simulink model "Adaptive_CT_ur10v"  (R2021b)
(part 18 of 20)

et24 = qd5.*(t1268.*-2.0-t1270.*2.0-t1739-t1742-t1788+t1823.*2.0+t1850-t1857-t1892+t2037+t2044+t2172+t2187+t2198+t2203+t8.*(t599+t612-t986-t1082-t1084+t449.*(t60-t190).*8.084033333333334e-4)+t2.*(t600+t610-t997-t1068-t1069+t451.*(t61-t239).*8.084033333333334e-4))-qd2.*(t2193+t2199+t1495.*t1680+t15.*t942.*t953+t17.*t942.*t953);
et25 = t1397-t1784-t1812+t1862+t1876-t1911-t1947-t2042-t2101+t2109+t2117+t2134+t2135-t2178+t2293+t2311+(t1321.*(t261+t455-t955-t1023))./2.0+t132.*(t600+t610-t997-t1068-t1069+t451.*(t61-t239).*8.084033333333334e-4)+t171.*(t599+t612-t986-t1082-t1084+t449.*(t60-t190).*8.084033333333334e-4);
et26 = t2.*t942.*(t441-t442-t647+t1012)+(t8.*t25.*(-t681+t1059.*(t61-t239).*8.084033333333334e-4+t341.*(t289-t476+t171.*(t60-t190)).*8.084033333333334e-4))./2.0;
et27 = (t8.*t29.*(t633-t852+t1418+t1752+t1545.*(t61-t239).*8.084033333333334e-4+t252.*(t289-t476+t171.*(t60-t190)).*8.084033333333334e-4))./2.0+t2.*t491.*(t426-t1001)+t8.*t491.*(t443-t1013);
et28 = t1546+t1549-t1588-t1988+t2063+t2072-t2139-t2141-t2176+t2225+t2283+t2286-t789.*t1680+(t25.*(t703+t979-t1289-t1291+t192.*(-t268-t292+t331+t334+t393+t2.*t25.*(t60-t190)).*8.084033333333334e-4+t236.*(-t267-t293+t348+t352+t382+t8.*t25.*(t61-t239)).*8.084033333333334e-4))./2.0;
et29 = t2.*t29.*(t599+t612-t986-t1082-t1084+t449.*(t60-t190).*8.084033333333334e-4)-t8.*t902.*t942-t2.*t914.*t942+(t8.*t25.*(t791+t1331+t935.*(t61-t239).*8.084033333333334e-4))./2.0;
et30 = t2331+qd4.*(t1643+t1644+t1732+t1782+t1841+t1843+t1991+t2001-t2008+t2035+t2041+t2171+t2183+t2196+t2202-t2223+t2275+t2279)+qd3.*(t1712+t1715+t1782+t1841+t1843+t1844+t2020+t2026+t2035+t2041-t2166+t2171+t2183+t2196+t2202+t2275+t2279);
et31 = -qd1.*(t713+t983-t1288-t1290-t1709+t1717-t2087-t2093+t192.*(-t268-t292+t331+t334+t393+t2.*t25.*(t60-t190)).*4.042016666666667e-4+t236.*(-t267-t293+t348+t352+t382+t8.*t25.*(t61-t239)).*4.042016666666667e-4)+qd2.*(t1739+t1742+t1782+t1841+t1843+t1892+t2040+t2046+t2171+t2185+t2196+t2202+t2275+t2279)+qd5.*(et28+et29);
et32 = t127+t220+t228+t255+t264-qd2.*(et23+et24)+qd3.*(-t2324+qd5.*(t1212+t1213+t1268+t1270+t1712+t1715+t1788+t1799+t1831+t1844+t1853+t1857+t2023+t2028+t2166+t2173+t2201+t2204+t2217+t2218)+qd4.*(t1428+t1430+t1434+t1436+t1454+t1458+t1884+t1923+t2151+t2152+t2193+t2199)+qd1.*(t540+t977+t1007+t1086+t1095-t1487+t1489+t1586+t1587)+qd2.*(t1507+t1513+t1514+t1515+t2080+t2083+t2193+t2199)+qd3.*(t2193+t2199+t1395.*t1680+t15.*t904.*t942+t17.*t904.*t942))+qdd3.*t2319+qdd4.*t2321;
et33 = qd6.*(t2328+qd2.*(t1710+t1719+t1783+t1789+t1840+t1859+t1969+t1975+t2030+t2170+t2205+t2210+t2306+t2310)+qd4.*(t1570+t1617+t1625+t1783+t1840+t1859-t1894+t1914+t1922+t1956+t1965+t2029+t2125+t2170+t2205+t2210+t2306+t2310)+qd1.*(t623+t778+t1383+t1390+t1670+t1721+t1735+t2021+t2025+(t915.*(t443-t1013))./2.0)-qd5.*(et25+et26+et27)+qd3.*(t1662+t1676+t1770+t1783+t1840+t1859+t1934+t1941+t1956+t1965+t1987+t2029+t2170+t2205+t2210+t2306+t2310))+qdd1.*(t542+t1077+t1105+t1591+t1592)+qdd2.*(t1821+t1822+t15.*t956+t17.*t956+t1680.^2);
et34 = -qd1.*(qd4.*(-t1304+t1306+t1424-t1427+t1537+t1540+t1955+t1959+t2165)+qd3.*(-t1465+t1468+t1487-t1489+t1586+t1587+t1955+t1959+t2165)-qd1.*(t243+t755+t757-t915.*t1099+t917.*t1101)+qd2.*(t1506+t1517+t1608+t1609+t1955+t1959+t2165)-qd6.*(t1218-t1433+t1554+t1670+t2000-t2002+t2021+t2025+(t915.*(t443-t1013))./2.0+(t29.*t30.*(t329+t834+t236.*(t61-t239).*8.084033333333334e-4))./2.0)+qd5.*(t1168+t1170+t1206+t1380+t1385+t1419+t1548+t1556+t1709+t1718+t1974+t1983+t2087+t2093+t2174));
et35 = qd4.*(qd3.*(t1426+t1429+t1435+t1437+t1454+t1458+t2126+t2149+t2151+t2193+t2199)+qd4.*(t1454+t1458+t1923+t2049+t2193+t2199-t1648.*t1792)+qd5.*(t1139+t1140+t1268+t1270+t1643+t1644+t1788+t1831+t1853+t1857+t1942+t1996+t2004+t2008+t2173+t2201+t2204+t2217+t2218+t2223)-qd6.*(t1617+t1625+t1790+t1856+t1861+t1894+t1913+t1921+t2124+t2175+t2209+t2212)+qd1.*(t540+t977+t1007+t1086+t1095-t1424+t1427+t1537+t1540)+qd2.*(t1463+t1467+t1469+t1470+t2155+t2157+t2193+t2199))+qdd6.*(t1683+t1700+t1785+t1869+t1871+t1900)-qdd5.*(t1726+t1728+t1786+t1842+t1846+t2018)-qd5.*(et30+et31);
et36 = t220-qdd1.*t981+qdd2.*t1802+qd2.*(t999+qd3.*(t452+t459-t1090-t1216+t15.*t20.*t22.*1.63763645e-1+t17.*t20.*t22.*1.63763645e-1)+qd2.*(t1066-t812.*(t2.*(t296-t2.*t9.*(1.53e+2./2.5e+2))+t8.*(t299-t8.*t9.*(1.53e+2./2.5e+2)))+t178.*t274+t179.*t274-t568.*t980))+qdd3.*(t211+t212+t15.*t31.*3.2752729e-1+t17.*t31.*3.2752729e-1+t980.^2);
et37 = qd3.*(t999+qd2.*(-t452-t459+t1090+t1216-t980.*(t2.*(t296-t2.*t9.*(1.53e+2./2.5e+2))+t8.*(t299-t8.*t9.*(1.53e+2./2.5e+2))).*2.0+t15.*t20.*t22.*4.91290935e-1+t17.*t20.*t22.*4.91290935e-1)+qd3.*(-t1193+t15.*t20.*t22.*3.2752729e-1+t17.*t20.*t22.*3.2752729e-1))-qd1.*(t1000+qd2.*t988-qd1.*(t151.*t400+t177.*t406));
et38 = t220+t229+qdd1.*t1532+qdd2.*t2177+qdd4.*t2179+qd2.*(-qd3.*(t752+t754+t1704-(t948.*t1138)./2.0+(t15.*t342.*t351)./2.0+(t17.*t342.*t351)./2.0)+qd1.*(t883-t889+t989+t990)+qd4.*(t506+t508+t596+t597+t1346+t1480-t1779+t1803+t15.*t144.*t342+t17.*t144.*t342)+qd2.*(t1108.*t1138+t15.*t342.*t420+t17.*t342.*t420))+qdd3.*(t519+t521+t15.*t356+t17.*t356+t1138.^2);
et39 = -qd3.*(qd4.*(-t506-t508-t1346.*2.0+t1737+t1808+t15.*t29.*t342.*1.22925e-1+t17.*t29.*t342.*1.22925e-1)-qd1.*t1945-qd2.*(t752+t754+t1704+t948.*t1138.*(3.0./2.0)-t15.*t342.*t351.*(3.0./2.0)-t17.*t342.*t351.*(3.0./2.0))+qd3.*(-t948.*t1138+t15.*t342.*t351+t17.*t342.*t351))-qd4.*(qd2.*(t495+t498+t506+t508+t596+t597+t1779+t1798+t1803)+qd4.*(t495+t498+t1352+t1627+t1165.*(t936-t937))+qd3.*(t496+t499+t506+t508+t1738+t1803)-qd1.*(-t661+t664+t1411))-qd1.*(qd1.*(t487+t502.*t708-t513.*t702)+qd3.*t1945+qd2.*(t882-t883+t889+t897+t989+t990)+qd4.*(t661-t664+t1411));
et40 = qd3.*(t1179+t1300-t1301-t1332+t1729+t1734-t1845+t2168-t2242+t2243+t25.*(t527+t813)+t2.*t29.*(t551-t821)+t8.*t29.*(t552-t822)+(t8.*t481.*(t423-t716))./2.0)-qd1.*(t710+t729-t830-t969+t991-t1173+t1508+t1874+(t836.*(t423-t716))./2.0+(t1100.*(t421-t432-t619+t718))./2.0)+qd4.*(t1179+t1261+t1267+t1300-t1301+t1673+t1674+t1720-t1733+t1916-t2162+t2224-t2242+t2243+t25.*(t527+t813)+t8.*t479.*(t421-t432-t619+t718)+t2.*t29.*(t551-t821)+t8.*t29.*(t552-t822));
et41 = qd2.*(t1179+t1300-t1301-t1332+t1720+t1756+t1759-t1845-t2162+t2186-t2242+t2243+t25.*(t527+t813)+t8.*t479.*(t421-t432-t619+t718)+t2.*t29.*(t551-t821)+t8.*t29.*(t552-t822)+(t8.*t481.*(t423-t716))./2.0)-qd5.*(t1147+t1153+t1361+t1479+t1484+t1593+t1707+t1771+t1773+t1837+t1839+t2073+t2231+t2247+t2248-t790.*t1603-t8.*t479.*t602+t2.*t479.*(t241-t419));
et42 = t220+t228+t256+t265-qd1.*(qd4.*(t527+t813+t952+t966+t1091-t1093+t1316+t1318+t1706+t1708)+qd1.*(t235+t525+t549-t829.*t1102+t836.*t1100)-qd3.*(t1159+t1166+t1169+t1384+t1386+t1705+t1711)-qd2.*(t1159+t1208+t1215-t1220+t1225+t1384+t1386+t1705+t1711)+qd5.*(t776+t787-t802+t806+t1070-t1131-t1187-t1189-t1251-t1252+t1508-t1724-t1725+t1874+(t836.*(t423-t716))./2.0+(t1100.*(t421-t432-t619+t718))./2.0))+qd5.*(et40+et41);
et43 = -qd3.*(qd2.*(t993+t995+t1202+t1211+t2084-t1396.*t1603.*(3.0./2.0)-t15.*t479.*t481.*(3.0./2.0)-t17.*t479.*t481.*(3.0./2.0))+qd4.*(t794.*(3.0./2.0)+t796.*(3.0./2.0)+t824+t826+t1202+t1211-t1885.*2.0+t2103+t2150)-qd5.*(t1192+t1201+t1234+t1236+t1313+t1320+t1332+t1333+t1456+t1457+t1730+t1731-t1797.*2.0+t1845+t2167+t6.*t15.*t130.*t479+t6.*t17.*t130.*t479)-qd3.*(t1203+t1209+t1396.*t1603+t15.*t479.*t481+t17.*t479.*t481)+qd1.*(t553+t798+t1166+t1169+t1384+t1386))+qdd2.*t2264+qdd4.*t2269;
et44 = qd2.*(qd3.*(t993+t995+t1203+t1209+t2084+(t1396.*t1603)./2.0+(t15.*t479.*t481)./2.0+(t17.*t479.*t481)./2.0)+qd5.*(t669+t672+t723+t726+t1192+t1201+t1234+t1236+t1313+t1320+t1332+t1333+t1456+t1457+t1756+t1759+t1800+t1832+t1845+t2186)-qd1.*(t553+t798-t1215+t1220+t1384+t1386)-qd4.*(t794+t796+t824+t826+t907+t908+t1202+t1211+t1886+t1925+t2133+t2150)+qd2.*(t1203+t1209+t1496.*t1603+t15.*t479.*t581+t17.*t479.*t581))+qdd3.*(t1277+t1278+t15.*t497+t17.*t497+t1603.^2)+qdd5.*(t1302-t1303-t1319-t1961+t25.*(t530-t803)+t8.*t479.*(t423-t716))+qdd1.*(t1160+t1353+t1358);
et45 = qd4.*(-qd4.*(t794+t796+t1202+t1211+t1886+t2052+t1535.*t1793)+qd5.*(t558+t560+t669+t672+t1192+t1201+t1234+t1236+t1271+t1275+t1313+t1320+t1456+t1457+t1673+t1674+t1800+t1916+t1943+t2224)+qd1.*(t540+t814-t1091+t1093+t1316+t1318)+qd2.*(-t794-t796+t824+t826+t907+t908+t1203+t1209-t2133+t2144+t2150)+qd3.*(t824-t825+t826-t827+t1203+t1209+t2103+t2150));
et46 = t1397-t1784-t1812+t1862+t1876-t1896-t1947-t2042+t2085-t2101+t2109+t2134+t2135-t2178+t2293+t2311+(t1321.*(t261+t455-t955-t1023))./2.0+t132.*(t600+t610-t997-t1068-t1069+t451.*(t61-t239).*8.084033333333334e-4)+t171.*(t599+t612-t986-t1082-t1084+t449.*(t60-t190).*8.084033333333334e-4);
et47 = t2.*t890.*(t441-t442-t647+t1012)+(t8.*t25.*(-t681+t1059.*(t61-t239).*8.084033333333334e-4+t341.*(t289-t476+t171.*(t60-t190)).*8.084033333333334e-4))./2.0;
et48 = (t8.*t29.*(t633-t852+t1418+t1752+t1545.*(t61-t239).*8.084033333333334e-4+t252.*(t289-t476+t171.*(t60-t190)).*8.084033333333334e-4))./2.0+t2.*t491.*(t426-t1001)+t8.*t491.*(t443-t1013);
et49 = t2324+qd2.*(t1507+t1514+t2083+t2194+t2197-t1395.*t1602.*(3.0./2.0)-t15.*t890.*t904.*(3.0./2.0)-t17.*t890.*t904.*(3.0./2.0))-qd1.*(t540+t977+t1007+t1086+t1095+t1441+t1445+t1586+t1587)+qd4.*(t1407.*(-3.0./2.0)-t1409.*(3.0./2.0)+t1426+t1429-t1884.*2.0+t2102+t2149+t2194+t2197)-qd3.*(t2193+t2199+t1395.*t1602+t15.*t890.*t904+t17.*t890.*t904);
et50 = qd5.*(t1212.*-2.0-t1213.*2.0-t1712-t1715-t1788+t1796.*2.0-t1844+t1850-t1857+t2020+t2026-t2166+t2172+t2198+t2203+t8.*(t599+t612-t986-t1082-t1084+t449.*(t60-t190).*8.084033333333334e-4)+t2.*(t600+t610-t997-t1068-t1069+t451.*(t61-t239).*8.084033333333334e-4));
et51 = t1546+t1549-t1588-t1988+t2063+t2072-t2139-t2141-t2176+t2225+t2283+t2286-t789.*t1602+(t25.*(t703+t979-t1289-t1291+t192.*(-t268-t292+t331+t334+t393+t2.*t25.*(t60-t190)).*8.084033333333334e-4+t236.*(-t267-t293+t348+t352+t382+t8.*t25.*(t61-t239)).*8.084033333333334e-4))./2.0;
et52 = t2.*t29.*(t599+t612-t986-t1082-t1084+t449.*(t60-t190).*8.084033333333334e-4)-t8.*t890.*t902-t2.*t890.*t914+(t8.*t25.*(t791+t1331+t935.*(t61-t239).*8.084033333333334e-4))./2.0;
et53 = t2331+qd4.*(t1643+t1644+t1732+t1782+t1841+t1843-t1915+t1991+t2001+t2014+t2024+t2161+t2171+t2196+t2202-t2223+t2275+t2279)-qd1.*(t713+t983-t1288-t1290-t1652+t1661-t2087-t2093+t192.*(-t268-t292+t331+t334+t393+t2.*t25.*(t60-t190)).*4.042016666666667e-4+t236.*(-t267-t293+t348+t352+t382+t8.*t25.*(t61-t239)).*4.042016666666667e-4);
et54 = qd3.*(t1712+t1715+t1782+t1841+t1843+t1844+t2023+t2028+t2166+t2171+t2196+t2202+t2275+t2279)+qd2.*(t1712+t1715+t1782+t1841+t1843+t1844+t2014+t2024+t2037+t2044+t2161+t2171+t2187+t2196+t2202+t2275+t2279)+qd5.*(et51+et52);
et55 = t220+t228+t255+t264+qdd2.*t2319+qdd4.*t2320+qd6.*(t2328+qd3.*(t1662+t1676+t1770+t1783+t1840+t1859+t1933+t1936+t1985+t2170+t2205+t2210+t2306+t2310)+qd4.*(t1570+t1617+t1625+t1783-t1814+t1840+t1859+t1914+t1922+t1930+t1931+t1977+t2125+t2170+t2205+t2210+t2306+t2310)+qd1.*(t623+t778+t1383+t1390+t1628+t1721+t1735+t2021+t2025+(t835.*(t443-t1013))./2.0)-qd5.*(et46+et47+et48)+qd2.*(t1662+t1676+t1770+t1783+t1840+t1859+t1930+t1931+t1973+t1977+t1980+t2032+t2170+t2205+t2210+t2306+t2310))-qd3.*(et49+et50);
et56 = qd2.*(qd3.*(t1507+t1514+t2083+t2193+t2199+(t1395.*t1602)./2.0+(t15.*t890.*t904)./2.0+(t17.*t890.*t904)./2.0)+qd5.*(t1212+t1213+t1268+t1270+t1712+t1715+t1788+t1799+t1831+t1844+t1853+t1857+t2040+t2046+t2173+t2185+t2201+t2204+t2217+t2218)+qd4.*(t1407+t1409+t1434+t1436+t1463+t1470+t1884+t1923+t2136+t2152+t2193+t2199)-qd6.*(t1662+t1676+t1770+t1790+t1856+t1861+t1969+t1975+t2030+t2175+t2209+t2212)+qd1.*(t540+t977+t1007+t1086+t1095-t1482+t1483+t1586+t1587)+qd2.*(t2193+t2199+t1495.*t1602+t15.*t890.*t953+t17.*t890.*t953))+qdd1.*(t542+t1077+t1105+t1572+t1573)+qdd3.*(t1821+t1822+t15.*t909+t17.*t909+t1602.^2);
et57 = -qd1.*(qd4.*(-t1246+t1247+t1348-t1350+t1537+t1540+t1955+t1959+t2165)+qd2.*(-t1476+t1478+t1482-t1483+t1586+t1587+t1955+t1959+t2165)-qd1.*(t243+t755+t757+t828.*t1101-t835.*t1099)+qd3.*(t1441+t1445+t1586+t1587+t1955+t1959+t2165)-qd6.*(t1218-t1433+t1554+t1628+t2000-t2002+t2021+t2025+(t835.*(t443-t1013))./2.0+(t29.*t30.*(t329+t834+t236.*(t61-t239).*8.084033333333334e-4))./2.0)+qd5.*(t1125+t1132+t1206+t1380+t1385+t1419+t1548+t1556+t1652+t1669+t1974+t1983+t2087+t2093+t2174))-qd5.*(et53+et54);
et58 = qd4.*(qd2.*(t1407+t1409+t1426+t1429+t1472+t1474+t2136+t2143+t2149+t2193+t2199)+qd4.*(t1407+t1409+t1884+t2049+t2193+t2199-t1534.*t1792)+qd5.*(t1139+t1140+t1212+t1213+t1643+t1644+t1788+t1799+t1853+t1857+t1915+t1942+t1996+t2004+t2173+t2201+t2204+t2217+t2218+t2223)-qd6.*(t1617+t1625+t1790+t1814+t1856+t1861+t1913+t1921+t2124+t2175+t2209+t2212)+qd1.*(t540+t977+t1007+t1086+t1095-t1348+t1350+t1537+t1540)+qd3.*(t1426+t1428+t1429+t1430+t2102+t2149+t2193+t2199))+qdd6.*(t1642+t1653+t1785+t1852+t1869+t1871)-qdd5.*(t1685+t1688+t1786+t1842+t1846+t1960);
et59 = t229+qdd1.*t1415+qdd3.*t2179+qdd2.*t2213-qd4.*(t1439+qd2.*(t346+t355-t586-t589+t1491+t1638-t1375.*(t936-t937).*2.0)+qd4.*(t1627+t15.*t25.*t29.*6.7158025e-3+t17.*t25.*t29.*6.7158025e-3)+qd3.*(t346+t355+t509+t512+t1357+t1638-t1165.*(t936-t937).*2.0))+qd2.*(t1432-qd4.*(t345+t354+t586+t589-t1491+t1633)-qd3.*(t505+t507+t509+t512+t586+t589+t1357+t1491+t1778+t1795)+qd2.*(t1485+t213.*t420+t214.*t420+t1274.*t1375+t1108.*(t936-t937)));
et60 = -qd1.*(qd1.*(t487-t25.*t744.*8.195e-2+t163.*t708)+qd4.*t1411+qd3.*(t663+t668+t1411)+qd2.*(t742+t768+t1411))+qdd4.*(t519+t521+(t936-t937).^2+t15.*t35.*6.7158025e-3+t17.*t35.*6.7158025e-3)-qd3.*(t1439+qd4.*(t345+t354+t496+t499-t1357+t1633)+qd3.*(t505+t507+t1346+t1795-t1138.*t1165)+qd2.*(t496+t499+t505+t507+t596+t597+t1357+t1491+t1795+t1798));
et61 = qd4.*(t1179+t1261+t1267+t1300-t1301+t1672+t1743-t2224-t2242+t2243+t25.*(t527+t813)+(t8.*t361.*(t421-t432-t619+t718))./2.0+t2.*t29.*(t551-t821)+t8.*t29.*(t552-t822))-qd1.*(t710+t729-t830-t969+t991-t1173+t1359+t1874+(t575.*(t423-t716))./2.0+(t1100.*(t421-t432-t619+t718))./2.0)+qd3.*(t1179+t1261+t1267+t1300-t1301+t1656+t1730+t1731+t1741-t1907+t2167-t2220-t2242+t2243+t25.*(t527+t813)+t8.*t361.*(t421-t432-t619+t718)+t2.*t29.*(t551-t821)+t8.*t29.*(t552-t822));
et62 = qd2.*(t1179+t1261+t1267+t1300-t1301+t1656+t1741+t1756+t1759-t2006+t2186-t2220-t2242+t2243+t25.*(t527+t813)+t8.*t361.*(t421-t432-t619+t718)+t2.*t29.*(t551-t821)+t8.*t29.*(t552-t822))-qd5.*(t1147+t1153+t1361+t1479+t1484+t1593+t1707+t1771+t1773+t1837+t1839+t2073+t2231+t2247+t2248-t790.*t1793-t8.*t361.*t602+t2.*t361.*(t241-t419));
et63 = t228+t256+t265-qd1.*(qd3.*(t527+t813+t974-t975+t1072+t1081+t1316+t1318+t1706+t1708)+qd2.*(t527+t813-t1031+t1038+t1141+t1146+t1316+t1318+t1706+t1708)+qd1.*(t235+t525+t549+t575.*t1100-t577.*t1102)+qd5.*(t679+t685-t802+t806+t1070-t1131-t1187-t1189-t1251-t1252+t1359-t1724-t1725+t1874+(t575.*(t423-t716))./2.0+(t1100.*(t421-t432-t619+t718))./2.0)+qd4.*(t527+t813+t887+t895+t1316+t1318+t1706+t1708))+qdd3.*t2269+qdd2.*t2300;
et64 = qd3.*(qd3.*(t793+t795+t1203+t1209+t1886+t2146+t1535.*t1603)+qd5.*(t558+t560+t669+t672+t1192+t1201+t1234+t1236+t1271+t1275+t1313+t1320+t1456+t1457+t1730+t1731+t1741+t1800+t1943+t2167)+qd1.*(t540+t814-t974+t975+t1316+t1318)+qd2.*(t793+t795+t837+t838+t907+t908+t1203+t1209+t1890+t1929+t2144+t2146)-qd4.*(t696+t698+t825+t827+t1202+t1211+t1890+t2057))+qdd4.*(t1277+t1278+t15.*t377+t17.*t377+t1793.^2)-qd4.*(qd4.*(t1202+t1211+t2052+t15.*t361.*t368+t17.*t361.*t368)-qd5.*(t1192+t1201+t1234+t1236+t1271+t1275+t1313+t1320+t1456+t1457+t1673+t1674+t1741-t1939.*2.0+t2224+t6.*t15.*t130.*t361+t6.*t17.*t130.*t361)+qd3.*(t697+t699-t825-t827+t1202+t1211+t1888+t2055-t1535.*t1793.*2.0)+qd2.*(t697+t699-t907-t908+t1202+t1211+t1927+t2055-t1649.*t1793.*2.0)-qd1.*(t540+t814+t887+t895+t1316+t1318));
et65 = qdd1.*(t1160+t1298+t1299)+qd5.*(et61+et62)+qd2.*(qd5.*(t558+t560+t723+t726+t1192+t1201+t1234+t1236+t1271+t1275+t1313+t1320+t1456+t1457+t1741+t1756+t1759+t1832+t1943+t2186)+qd1.*(t540+t814+t1031-t1038+t1316+t1318)+qd2.*(t1203+t1209+t1925+t1496.*t1793+t1649.*t1681+t15.*t361.*t581+t17.*t361.*t581)+qd3.*(t793+t795+t825+t827+t911+t912+t1203+t1209+t1890+t1929+t2127+t2146)-qd4.*(t696+t698+t907+t908+t1202+t1211+t1929+t2057))-qdd5.*(t1178+t1239+t1244+t1303+t1309+t2119);
et66 = t1397-t1784-t1812+t1862-t1868+t1876-t1947-t2042-t2101+t2109+t2134+t2135+t2159-t2178+t2293+t2311+(t1321.*(t261+t455-t955-t1023))./2.0+t132.*(t600+t610-t997-t1068-t1069+t451.*(t61-t239).*8.084033333333334e-4)+t171.*(t599+t612-t986-t1082-t1084+t449.*(t60-t190).*8.084033333333334e-4);
et67 = t2.*t773.*(t441-t442-t647+t1012)+(t8.*t25.*(-t681+t1059.*(t61-t239).*8.084033333333334e-4+t341.*(t289-t476+t171.*(t60-t190)).*8.084033333333334e-4))./2.0;
et68 = (t8.*t29.*(t633-t852+t1418+t1752+t1545.*(t61-t239).*8.084033333333334e-4+t252.*(t289-t476+t171.*(t60-t190)).*8.084033333333334e-4))./2.0+t2.*t491.*(t426-t1001)+t8.*t491.*(t443-t1013);
et69 = t2327-qd4.*(t1576+t1617+t1625+t1783+t1840+t1859+t1913+t1921+t2124+t2170+t2205+t2210+t2306+t2310)+qd3.*(t1576-t1783-t1811-t1840+t1854-t1905+t1933+t1936+t1985-t2123-t2170-t2205+t2208+t2304+t2308+t8.*t773.*(t261+t455-t955-t1023)+(t2.*t785.*(t426-t1001))./2.0+(t8.*t785.*(t443-t1013))./2.0)+qd2.*(t1576-t1783-t1840+t1854-t1891-t1905+t1969+t1975+t2030-t2123-t2170-t2205+t2208+t2304+t2308+t8.*t773.*(t261+t455-t955-t1023)+(t2.*t785.*(t426-t1001))./2.0+(t8.*t785.*(t443-t1013))./2.0)-qd1.*(t623+t778+t1383+t1390+t1538+t1721+t1735+t2021+t2025+(t574.*(t443-t1013))./2.0);
et70 = qd5.*(et66+et67+et68);
et71 = t1546+t1549-t1588-t1988+t2063+t2072-t2139-t2141-t2176+t2225+t2283+t2286-t789.*t1792+(t25.*(t703+t979-t1289-t1291+t192.*(-t268-t292+t331+t334+t393+t2.*t25.*(t60-t190)).*8.084033333333334e-4+t236.*(-t267-t293+t348+t352+t382+t8.*t25.*(t61-t239)).*8.084033333333334e-4))./2.0;
et72 = t2.*t29.*(t599+t612-t986-t1082-t1084+t449.*(t60-t190).*8.084033333333334e-4)-t8.*t773.*t902-t2.*t773.*t914+(t8.*t25.*(t791+t1331+t935.*(t61-t239).*8.084033333333334e-4))./2.0;
et73 = t2331+qd3.*(t1643+t1644-t1740+t1782+t1841+t1843+t1906+t1989+t1999+t2020+t2026-t2166+t2171+t2196+t2202+t2219+t2275+t2279)-qd1.*(t713+t983-t1288-t1290-t1574+t1580-t2087-t2093+t192.*(-t268-t292+t331+t334+t393+t2.*t25.*(t60-t190)).*4.042016666666667e-4+t236.*(-t267-t293+t348+t352+t382+t8.*t25.*(t61-t239)).*4.042016666666667e-4);
et74 = qd4.*(t1643+t1644+t1740+t1782+t1841+t1843+t1996+t2004+t2171+t2196+t2202+t2223+t2275+t2279)+qd2.*(t1643+t1644-t1740+t1782+t1841+t1843+t1989+t1999+t2005+t2037+t2044+t2171+t2187+t2196+t2202+t2219+t2275+t2279)+qd5.*(et71+et72);
et75 = -qd4.*(t2049+t2193+t2199+t15.*t773.*t785+t17.*t773.*t785)+qd3.*(t1343+t1344+t1428+t1430+t1887+t2054+t2194+t2197-t1534.*t1792.*2.0)+qd2.*(t1343+t1344+t1463+t1470+t1926+t2054+t2194+t2197-t1648.*t1792.*2.0);
et76 = qd5.*(t1139.*-2.0-t1140.*2.0+t1646+t1650-t1740-t1788+t1850-t1857+t1938.*2.0+t1991+t2001+t2172+t2198+t2203-t2223+t8.*(t599+t612-t986-t1082-t1084+t449.*(t60-t190).*8.084033333333334e-4)+t2.*(t600+t610-t997-t1068-t1069+t451.*(t61-t239).*8.084033333333334e-4))-qd1.*(t540+t977+t1007+t1086+t1095+t1176+t1181+t1537+t1540);
et77 = qd6.*(t1576+t1617+t1625+t1790+t1856+t1861+t1913+t1921+t2124+t2175+t2209+t2212);
et78 = t228+t255+t264-qd6.*(et69+et70)+qd2.*(qd5.*(t1139+t1140+t1268+t1270+t1643+t1644+t1740+t1788+t1831+t1853+t1857+t1942+t2040+t2046+t2173+t2185+t2201+t2204+t2217+t2218)+qd3.*(t1405+t1408+t1435+t1437+t1463+t1470+t1889+t1928+t2126+t2145+t2193+t2199)-qd6.*(t1576+t1617+t1625+t1790+t1856+t1861+t1969+t1975+t2030+t2175+t2209+t2212)+qd1.*(t540+t977+t1007+t1086+t1095-t1315+t1317+t1537+t1540)+qd4.*(t1339+t1341+t1463+t1470+t1926+t2054+t2193+t2199)+qd2.*(-t1923+t2193+t2199+t1495.*t1792+t1648.*t1680+t15.*t773.*t953+t17.*t773.*t953))+qdd2.*t2321+qdd3.*t2320-qd5.*(et73+et74)+qdd1.*(t542+t1077+t1105+t1522+t1523)+qdd4.*(t1821+t1822+t15.*t777+t17.*t777+t1792.^2);
et79 = -qd1.*(qd3.*(t1262-t1265-t1337+t1338+t1537+t1540+t1955+t1959+t2165)+qd2.*(t1315-t1317-t1402+t1406+t1537+t1540+t1955+t1959+t2165)-qd1.*(t243+t755+t757-t574.*t1099+t576.*t1101)+qd4.*(t1176+t1181+t1537+t1540+t1955+t1959+t2165)-qd6.*(t1218-t1433+t1538+t1554+t2000-t2002+t2021+t2025+(t574.*(t443-t1013))./2.0+(t29.*t30.*(t329+t834+t236.*(t61-t239).*8.084033333333334e-4))./2.0)+qd5.*(t1039+t1049+t1206+t1380+t1385+t1419+t1548+t1556+t1574+t1582+t1974+t1983+t2087+t2093+t2174))-qd4.*(et75+et76+et77);
et80 = qd3.*(qd5.*(t1139+t1140+t1212+t1213+t1643+t1644+t1740+t1788+t1799+t1853+t1857+t1942+t2023+t2028+t2166+t2173+t2201+t2204+t2217+t2218)+qd3.*(t1405+t1408-t1884+t2145+t2193+t2199+t1534.*t1602)+qd2.*(t1405+t1408+t1428+t1430+t1472+t1474+t1889+t1928+t2143+t2145+t2193+t2199)-qd6.*(t1576+t1617+t1625+t1790+t1856+t1861+t1933+t1936+t1985+t2175+t2209+t2212)+qd1.*(t540+t977+t1007+t1086+t1095-t1262+t1265+t1537+t1540)+qd4.*(t1339+t1341+t1428+t1430+t1887+t2054+t2193+t2199))+qdd6.*(t1610+t1616+t1785+t1869+t1871+t2013)-qdd5.*(t1631+t1634+t1786+t1842+t1846+t2118);
et81 = qd4.*(-t919+t1148+t1154+t1599+t1613+t1615+t1692+t1766+t1767+t1838+t1849-t1979+t2075+t2227+t2245+t2246+(t2.*t361.*(t241-t419))./2.0)+qd3.*(-t1003+t1148+t1154+t1599+t1613+t1615+t1692+t1766+t1767-t1817+t1838+t1849+t2075+t2227+t2245+t2246+(t2.*t479.*(t241-t419))./2.0)+qd2.*(-t1065+t1148+t1154+t1599+t1613+t1615+t1692+t1766+t1767+t1838+t1849-t1865+t2075+t2227+t2245+t2246+(t2.*t580.*(t241-t419))./2.0);
et82 = -qd1.*(t1256+t1259+t1452+t1461+t6.*t29.*t624.*5.077704166666666e-4+t12.*t29.*t622.*5.077704166666666e-4)+qd5.*(t25.*(t972+t973).*(-1.0./2.0)-t790.*t1264+t1036.*(t241-t419)+t602.*(t423-t716)+(t8.*t29.*t1597)./2.0+(t2.*t29.*(t1026-t1043))./2.0);
et83 = qd1.*(t12.*t68.*1.015540833333333e-3+t371.*t1100+t380.*t1102)+qd5.*(t972+t973+t1256+t1259+t1452+t1461-t12.*t25.*t68.*1.015540833333333e-3+(t2.*t29.*t1097)./2.0+(t8.*t29.*(t614-t638))./2.0)+qd4.*(t693+t695+t711+t712-t831-t970+t982+t1129+t1130-t1174+t1196+t1198+t1349+t1863+t575.*(t423-t716)+t1100.*(t421-t432-t619+t718))-qd3.*(-t809-t818+t1133+t1134+t1188+t1190+t1502+t1505+t1866+t1872+t2216);
et84 = -qd2.*(-t891-t898+t1133+t1134+t1188+t1190+t1551+t1553+t1866+t1872+t2216);
et85 = -qd4.*(qd4.*(t558+t560+t1255+t1260+t1464+t1466+t1659+t1668+t1733+t1943+t2220+t2240+t2241)-qd5.*(t919+t924+t1157+t1161+t1379+t1490+t1492+t1595+t1611+t1612+t1979)+qd3.*(t559+t561+t670+t673+t1255+t1260+t1464+t1466+t1659+t1668+t1810+t1907+t1954+t2220+t2240+t2241)+qd2.*(t559+t561+t724+t727+t1255+t1260+t1464+t1466+t1659+t1668+t1848+t1954+t2006+t2220+t2240+t2241)-qd1.*(t693+t695+t805+t815+t1196+t1198))-qd3.*(qd3.*(t669+t672+t1323+t1325+t1464+t1466+t1723+t1727+t1800+t1826+t2162+t2240+t2241)-qd5.*(t1003+t1015+t1157+t1161+t1379+t1490+t1492+t1595+t1611+t1612+t1817)+qd4.*(t559+t561+t670+t673+t1255+t1260+t1464+t1466+t1723+t1727+t1733+t1810+t1954+t2162+t2240+t2241)+qd2.*(t670+t673+t724+t727+t1323+t1325+t1464+t1466+t1723+t1727+t1810+t1826+t1848+t2162+t2240+t2241)-qd1.*(t805+t809+t815+t818+t1196+t1198))-t6.*t29.*5.675085e-1;
et86 = -qdd3.*(t1319+t1322+t1748+t1757+t1961)-qdd4.*(t1239+t1244+t1748+t1757+t2119)-qdd2.*(t1356+t1360+t1748+t1757+t2019)-qdd1.*(t1620+t1623+t1658)+qdd5.*((t423-t716).^2+t25.*t1658+t1036.^2+t1264.^2+t2.*t29.*t1744+t8.*t29.*t1745)+qd5.*(et81+et82)-qd2.*(qd1.*(t801-t805-t891-t898+t1188+t1190)-qd5.*(t1065+t1078+t1157+t1161+t1379+t1490+t1492+t1595+t1611+t1612+t1865)+qd4.*(t559+t561+t724+t727+t1255+t1260+t1464+t1466+t1733+t1747+t1750+t1848+t1954+t2184+t2240+t2241)+qd3.*(t670+t673+t724+t727+t1323+t1325+t1464+t1466+t1747+t1750+t1810+t1826+t1848+t2184+t2240+t2241)+qd2.*(t723+t726+t1464+t1466+t1747+t1750+t1832+t2184+t2240+t2241+t1264.*t1496+t2.*t581.*t1036-t8.*t581.*(t423-t716)))+qd1.*(et83+et84);
et87 = qd6.*(t1416-t1791+t1873-t1880+t1882+t2163-t2182+(t132.*(t600+t610-t997-t1068-t1069+t451.*(t61-t239).*8.084033333333334e-4))./2.0+(t171.*(t599+t612-t986-t1082-t1084+t449.*(t60-t190).*8.084033333333334e-4))./2.0+(t2.*t773.*(t441-t442-t647+t1012))./2.0+(t2.*t491.*(t426-t1001))./2.0+(t8.*t491.*(t443-t1013))./2.0);
et88 = -1.0;
et89 = qd6.*(t1416-t1791+t1873+t1882-t1898+t2090-t2182+(t132.*(t600+t610-t997-t1068-t1069+t451.*(t61-t239).*8.084033333333334e-4))./2.0+(t171.*(t599+t612-t986-t1082-t1084+t449.*(t60-t190).*8.084033333333334e-4))./2.0+(t2.*t890.*(t441-t442-t647+t1012))./2.0+(t2.*t491.*(t426-t1001))./2.0+(t8.*t491.*(t443-t1013))./2.0);
et90 = -1.0;
et91 = qd5.*(t1500+t1511+t1563+t1567+t1594+t1864+t2181+t2229+t2232+t2252+t2253);
et92 = qd6.*(t1416-t1791+t1873+t1882-t1920+t2121-t2182+(t132.*(t600+t610-t997-t1068-t1069+t451.*(t61-t239).*8.084033333333334e-4))./2.0+(t171.*(t599+t612-t986-t1082-t1084+t449.*(t60-t190).*8.084033333333334e-4))./2.0+(t2.*t942.*(t441-t442-t647+t1012))./2.0+(t2.*t491.*(t426-t1001))./2.0+(t8.*t491.*(t443-t1013))./2.0);
et93 = -qd4.*(t1152+t1155+t1284+t1286+t1639+t1640+t1732+t1847+t1953+t2035+t2041+t2183+t2221+t2222+t2273+t2274)-qd3.*(t1228+t1229+t1284+t1286+t1693+t1701+t1809+t1825+t1847+t2035+t2041+t2183+t2221+t2222+t2273+t2274)-qd2.*(t1268+t1270+t1831+t2035+t2041+t2183+t2221+t2222+t2273+t2274+t1263.*t1495+t2.*t953.*t1314+t8.*t953.*t1321)+qd1.*(t541+t554+t926+t932+t1016+t1018+t1180+t1182+t1399+t1400);
et94 = t1455+t1664+t1665+t1901+t2058+t2064+t6.*t1982-t133.*t2034-(t25.*t2256)./2.0+t132.*t2251+t170.*(t791+t1331+t935.*(t61-t239).*8.084033333333334e-4)-t171.*(t784-t804-t1142+t1280-t1293+t665.*(t60-t190).*8.084033333333334e-4);
et95 = (t2.*t29.*(t682+t941-t1378-t1624+t1370.*(t60-t190).*8.084033333333334e-4+t7.*t171.*(t289-t476+t171.*(t60-t190)).*8.084033333333334e-4))./2.0;
et96 = t8.*t29.*(t691+t934-t1367-t1630+t1371.*(t61-t239).*8.084033333333334e-4+t7.*t132.*(t289-t476+t171.*(t60-t190)).*8.084033333333334e-4).*(-1.0./2.0)+t12.*t29.*t2249;
et97 = t1964+t1966+t192.*t1370.*4.042016666666667e-4-t236.*t1371.*4.042016666666667e-4+(t378.*(t426-t1001))./2.0+(t370.*(t443-t1013))./2.0+t12.*t39.*(t289-t476+t171.*(t60-t190)).*4.042016666666667e-4-(t6.*t29.*t486)./1.0e+4+(t12.*t29.*t774)./1.0e+4;
et98 = t12.*t40.*t1059.*(-4.042016666666667e-4);
et99 = t1416-t1804-t1880-t1937+t1986+t2059-t2097+t2128+t2129+t2163+t2291-t2292+(t8.*(t682+t941-t1378-t1624+t1370.*(t60-t190).*8.084033333333334e-4+t7.*t171.*(t289-t476+t171.*(t60-t190)).*8.084033333333334e-4))./2.0;
et100 = (t2.*(t691+t934-t1367-t1630+t1371.*(t61-t239).*8.084033333333334e-4+t7.*t132.*(t289-t476+t171.*(t60-t190)).*8.084033333333334e-4))./2.0+t1321.*(t261+t455-t955-t1023);
et101 = t12.*t29.*(t703+t979-t1289-t1291+t192.*(-t268-t292+t331+t334+t393+t2.*t25.*(t60-t190)).*8.084033333333334e-4+t236.*(-t267-t293+t348+t352+t382+t8.*t25.*(t61-t239)).*8.084033333333334e-4)+(t2.*t773.*(t441-t442-t647+t1012))./2.0;
et102 = t29.*t30.*(t791+t1331+t935.*(t61-t239).*8.084033333333334e-4)+(t2.*t491.*(t426-t1001))./2.0+(t8.*t491.*(t443-t1013))./2.0;
et103 = t1416-t1804-t1898-t1937+t1986+t2059+t2090-t2097+t2128+t2129+t2291-t2292+(t8.*(t682+t941-t1378-t1624+t1370.*(t60-t190).*8.084033333333334e-4+t7.*t171.*(t289-t476+t171.*(t60-t190)).*8.084033333333334e-4))./2.0;
et104 = (t2.*(t691+t934-t1367-t1630+t1371.*(t61-t239).*8.084033333333334e-4+t7.*t132.*(t289-t476+t171.*(t60-t190)).*8.084033333333334e-4))./2.0+t1321.*(t261+t455-t955-t1023);
et105 = t12.*t29.*(t703+t979-t1289-t1291+t192.*(-t268-t292+t331+t334+t393+t2.*t25.*(t60-t190)).*8.084033333333334e-4+t236.*(-t267-t293+t348+t352+t382+t8.*t25.*(t61-t239)).*8.084033333333334e-4)+(t2.*t890.*(t441-t442-t647+t1012))./2.0;
et106 = t29.*t30.*(t791+t1331+t935.*(t61-t239).*8.084033333333334e-4)+(t2.*t491.*(t426-t1001))./2.0+(t8.*t491.*(t443-t1013))./2.0;
et107 = t1416-t1804-t1920-t1937+t1986+t2059-t2097+t2121+t2128+t2129+t2291-t2292+(t8.*(t682+t941-t1378-t1624+t1370.*(t60-t190).*8.084033333333334e-4+t7.*t171.*(t289-t476+t171.*(t60-t190)).*8.084033333333334e-4))./2.0;
et108 = (t2.*(t691+t934-t1367-t1630+t1371.*(t61-t239).*8.084033333333334e-4+t7.*t132.*(t289-t476+t171.*(t60-t190)).*8.084033333333334e-4))./2.0+t1321.*(t261+t455-t955-t1023);
et109 = t12.*t29.*(t703+t979-t1289-t1291+t192.*(-t268-t292+t331+t334+t393+t2.*t25.*(t60-t190)).*8.084033333333334e-4+t236.*(-t267-t293+t348+t352+t382+t8.*t25.*(t61-t239)).*8.084033333333334e-4)+(t2.*t942.*(t441-t442-t647+t1012))./2.0;
et110 = t29.*t30.*(t791+t1331+t935.*(t61-t239).*8.084033333333334e-4)+(t2.*t491.*(t426-t1001))./2.0+(t8.*t491.*(t443-t1013))./2.0;
et111 = (t132.*(t691+t934-t1367-t1630+t1371.*(t61-t239).*8.084033333333334e-4+t7.*t132.*(t289-t476+t171.*(t60-t190)).*8.084033333333334e-4))./2.0;
et112 = (t171.*(t682+t941-t1378-t1624+t1370.*(t60-t190).*8.084033333333334e-4+t7.*t171.*(t289-t476+t171.*(t60-t190)).*8.084033333333334e-4))./2.0-(t6.*t2033)./2.0+(t133.*t2094)./2.0+t943.*t1503+t1695.*(t443-t1013)-(t426-t1001).*(t441-t442-t647+t1012);
et113 = t170.*(-t681+t1059.*(t61-t239).*8.084033333333334e-4+t341.*(t289-t476+t171.*(t60-t190)).*8.084033333333334e-4).*(-1.0./2.0)-(t12.*t29.*t2256)./2.0;
et114 = t1497+t1498+t1578+t1585+t192.*t665.*4.042016666666667e-4-t236.*t666.*4.042016666666667e-4-(t6.*t29.*t624)./1.0e+4-(t12.*t29.*t622)./1.0e+4+t12.*t39.*t923.*4.042016666666667e-4;
et115 = t12.*t40.*t935.*(-4.042016666666667e-4);
et116 = -t1475-t1486+t1560+t1562-t1594-t1816-t1982+t2053+t2074-t2140-t2142-t2255+t2277+t2281+t25.*(t703+t979-t1289-t1291+t192.*(-t268-t292+t331+t334+t393+t2.*t25.*(t60-t190)).*8.084033333333334e-4+t236.*(-t267-t293+t348+t352+t382+t8.*t25.*(t61-t239)).*8.084033333333334e-4);
et117 = (t8.*(t784-t804-t1142+t1280-t1293+t665.*(t60-t190).*8.084033333333334e-4))./2.0+t8.*t25.*(t791+t1331+t935.*(t61-t239).*8.084033333333334e-4);
et118 = -t1401-t1422+t1560+t1562-t1594-t1978-t1982+t2053+t2074-t2140-t2142-t2255+t2277+t2281+t25.*(t703+t979-t1289-t1291+t192.*(-t268-t292+t331+t334+t393+t2.*t25.*(t60-t190)).*8.084033333333334e-4+t236.*(-t267-t293+t348+t352+t382+t8.*t25.*(t61-t239)).*8.084033333333334e-4);
et119 = (t8.*(t784-t804-t1142+t1280-t1293+t665.*(t60-t190).*8.084033333333334e-4))./2.0+t8.*t25.*(t791+t1331+t935.*(t61-t239).*8.084033333333334e-4);
et120 = -t1500-t1511+t1560+t1562-t1594-t1864-t1982+t2053+t2074-t2140-t2142-t2255+t2277+t2281+t25.*(t703+t979-t1289-t1291+t192.*(-t268-t292+t331+t334+t393+t2.*t25.*(t60-t190)).*8.084033333333334e-4+t236.*(-t267-t293+t348+t352+t382+t8.*t25.*(t61-t239)).*8.084033333333334e-4);
et121 = (t8.*(t784-t804-t1142+t1280-t1293+t665.*(t60-t190).*8.084033333333334e-4))./2.0+t8.*t25.*(t791+t1331+t935.*(t61-t239).*8.084033333333334e-4);
et122 = qd5.*(t789.*t1263+t902.*t1321+t914.*t1314-(t25.*t2249)./2.0+(t2.*t29.*(t784-t804-t1142+t1280-t1293+t665.*(t60-t190).*8.084033333333334e-4))./2.0+(t8.*t29.*t2251)./2.0)+qd1.*(et114+et115);
et123 = qd6.*(t1455+t1664+t1665+t1901+t2058+t2064+t6.*t1988-(t133.*t2034)./2.0+(t132.*t2251)./2.0+(t170.*(t791+t1331+t935.*(t61-t239).*8.084033333333334e-4))./2.0-(t171.*(t784-t804-t1142+t1280-t1293+t665.*(t60-t190).*8.084033333333334e-4))./2.0+(t12.*t29.*t2249)./2.0)-qd3.*(et116+et117)-qd4.*(et118+et119)-qd2.*(et120+et121);
et124 = t703+t979-t1057-t1062-t1289-t1291+t1388+t1394-t1568+t1571-t1918-t2082-t2086+t192.*(-t268-t292+t331+t334+t393+t2.*t25.*(t60-t190)).*8.084033333333334e-4+t236.*(-t267-t293+t348+t352+t382+t8.*t25.*(t61-t239)).*8.084033333333334e-4;
et125 = (t8.*(t324-t344+t730-t731-t765+t12.*t39.*(t60-t190).*8.084033333333334e-4))./2.0;
et126 = t703+t979-t1135-t1143-t1289-t1291+t1388+t1394-t1641+t1645-t1918-t2082-t2086+t192.*(-t268-t292+t331+t334+t393+t2.*t25.*(t60-t190)).*8.084033333333334e-4+t236.*(-t267-t293+t348+t352+t382+t8.*t25.*(t61-t239)).*8.084033333333334e-4;
et127 = (t8.*(t324-t344+t730-t731-t765+t12.*t39.*(t60-t190).*8.084033333333334e-4))./2.0;
et128 = t703+t979-t1180-t1182-t1289-t1291+t1388+t1394-t1691+t1703-t1918-t2082-t2086+t192.*(-t268-t292+t331+t334+t393+t2.*t25.*(t60-t190)).*8.084033333333334e-4+t236.*(-t267-t293+t348+t352+t382+t8.*t25.*(t61-t239)).*8.084033333333334e-4;
et129 = (t8.*(t324-t344+t730-t731-t765+t12.*t39.*(t60-t190).*8.084033333333334e-4))./2.0;
et130 = -qd1.*(t12.*t68.*(-2.0e-4)+t370.*t1099+t378.*t1101+t12.*t39.*t192.*8.084033333333334e-4-t12.*t40.*t236.*8.084033333333334e-4)+qd4.*(et124+et125)+qd3.*(et126+et127)+qd2.*(et128+et129);
et131 = qd6.*(t1964+t1966-(t6.*t1185)./2.0+(t133.*t1501)./2.0-(t132.*t1904)./2.0+(t171.*(t324-t344+t730-t731-t765+t12.*t39.*(t60-t190).*8.084033333333334e-4))./2.0-(t170.*(t329+t834+t236.*(t61-t239).*8.084033333333334e-4))./2.0+(t378.*(t426-t1001))./2.0+(t370.*(t443-t1013))./2.0-(t12.*t29.*t1242)./2.0);
et132 = -qd5.*(-t704-t705+t1083-t1103+t1217-t1226+t1497+t1498+t1578+t1585+(t25.*t1242)./2.0-(t8.*t29.*t1904)./2.0-(t2.*t29.*(t324-t344+t730-t731-t765+t12.*t39.*(t60-t190).*8.084033333333334e-4))./2.0);
et133 = -qd4.*(qd4.*(t1139+t1140+t1639+t1640+t1732+t1942+t1989+t1999+t2219+t2221+t2222+t2273+t2274)+et87.*et88-qd5.*(t1401+t1422+t1563+t1567+t1594+t1978+t2181+t2229+t2232+t2252+t2253)+qd3.*(t1152+t1155+t1228+t1229+t1639+t1640+t1809+t1906+t1953+t1989+t1999+t2219+t2221+t2222+t2273+t2274)+qd2.*(t1152+t1155+t1284+t1286+t1639+t1640+t1847+t1953+t1989+t1999+t2005+t2219+t2221+t2222+t2273+t2274)-qd1.*(t541+t554+t926+t932+t1016+t1018+t1057+t1062+t1399+t1400))-qd3.*(qd3.*(t1212+t1213+t1693+t1701+t1799+t1825+t2014+t2024+t2161+t2221+t2222+t2273+t2274)-qd5.*(t1475+t1486+t1563+t1567+t1594+t1816+t2181+t2229+t2232+t2252+t2253)+et89.*et90+qd4.*(t1152+t1155+t1228+t1229+t1639+t1640+t1732+t1809+t1953+t2014+t2024+t2161+t2221+t2222+t2273+t2274)+qd2.*(t1228+t1229+t1284+t1286+t1693+t1701+t1809+t1825+t1847+t2014+t2024+t2161+t2221+t2222+t2273+t2274)-qd1.*(t541+t554+t926+t932+t1016+t1018+t1135+t1143+t1399+t1400));
et134 = t6.*t29.*(-1.356723)-qdd3.*(t1685+t1688+t1960+t2047+t2051)-qdd4.*(t1631+t1634+t2047+t2051+t2118)-qdd2.*(t1726+t1728+t2018+t2047+t2051)+qdd5.*(t25.*t1963+t1263.^2+t1314.^2+t1321.^2+t2.*t29.*t2034+t8.*t29.*(t791+t1331+t935.*(t61-t239).*8.084033333333334e-4))-qdd1.*(t1775+t1776+t1963)+qd2.*(et91+et92+et93)+qd6.*(qd5.*(et94+et95+et96)-qd1.*(et97+et98)+qd4.*(et99+et100+et101+et102)+qd3.*(et103+et104+et105+et106)+qd2.*(et107+et108+et109+et110)+qd6.*(et111+et112+et113));
et135 = qdd6.*(-t1679+t12.*t1982+t171.*t2034-t132.*(t791+t1331+t935.*(t61-t239).*8.084033333333334e-4)+t1314.*(t426-t1001)+t1321.*(t443-t1013))-qd5.*(et122+et123)-qd1.*(et130+et131+et132);
et136 = t789.*t943+t25.*t2256+t1263.*t1503-t1321.*t1695-t914.*(t426-t1001)-t902.*(t443-t1013)+t1314.*(t441-t442-t647+t1012)-t2.*t29.*(t682+t941-t1378-t1624+t1370.*(t60-t190).*8.084033333333334e-4+t7.*t171.*(t289-t476+t171.*(t60-t190)).*8.084033333333334e-4);
et137 = t8.*t29.*(t691+t934-t1367-t1630+t1371.*(t61-t239).*8.084033333333334e-4+t7.*t132.*(t289-t476+t171.*(t60-t190)).*8.084033333333334e-4);
et138 = t132.*(t691+t934-t1367-t1630+t1371.*(t61-t239).*8.084033333333334e-4+t7.*t132.*(t289-t476+t171.*(t60-t190)).*8.084033333333334e-4);
et139 = t171.*(t682+t941-t1378-t1624+t1370.*(t60-t190).*8.084033333333334e-4+t7.*t171.*(t289-t476+t171.*(t60-t190)).*8.084033333333334e-4)-t6.*t2033+t133.*t2094+t943.*t1503.*2.0+t1695.*(t443-t1013).*2.0-(t426-t1001).*(t441-t442-t647+t1012).*2.0;
et140 = -t170.*(-t681+t1059.*(t61-t239).*8.084033333333334e-4+t341.*(t289-t476+t171.*(t60-t190)).*8.084033333333334e-4)-t12.*t29.*t2256;
et141 = t1397-t1911+t2117+t8.*(t682+t941-t1378-t1624+t1370.*(t60-t190).*8.084033333333334e-4+t7.*t171.*(t289-t476+t171.*(t60-t190)).*8.084033333333334e-4);
et142 = t2.*(t691+t934-t1367-t1630+t1371.*(t61-t239).*8.084033333333334e-4+t7.*t132.*(t289-t476+t171.*(t60-t190)).*8.084033333333334e-4)+t2.*t942.*(t441-t442-t647+t1012)+t2.*t491.*(t426-t1001)+t8.*t491.*(t443-t1013);
et143 = t1397-t1896+t2085+t8.*(t682+t941-t1378-t1624+t1370.*(t60-t190).*8.084033333333334e-4+t7.*t171.*(t289-t476+t171.*(t60-t190)).*8.084033333333334e-4);
et144 = t2.*(t691+t934-t1367-t1630+t1371.*(t61-t239).*8.084033333333334e-4+t7.*t132.*(t289-t476+t171.*(t60-t190)).*8.084033333333334e-4)+t2.*t890.*(t441-t442-t647+t1012)+t2.*t491.*(t426-t1001)+t8.*t491.*(t443-t1013);
et145 = t1397-t1868+t2159+t8.*(t682+t941-t1378-t1624+t1370.*(t60-t190).*8.084033333333334e-4+t7.*t171.*(t289-t476+t171.*(t60-t190)).*8.084033333333334e-4);
et146 = t2.*(t691+t934-t1367-t1630+t1371.*(t61-t239).*8.084033333333334e-4+t7.*t132.*(t289-t476+t171.*(t60-t190)).*8.084033333333334e-4)+t2.*t773.*(t441-t442-t647+t1012)+t2.*t491.*(t426-t1001)+t8.*t491.*(t443-t1013);
et147 = -qd1.*(qd4.*(t1528+t2012+t2017+t2282+t574.*(t443-t1013))+qd3.*(t1619+t2012+t2017+t2282+t835.*(t443-t1013))+qd2.*(t1651+t2012+t2017+t2282+t915.*(t443-t1013))-qd5.*(-t608+t888-t1328+t1596-t1601+t1951+t1952+t378.*(t426-t1001)+t370.*(t443-t1013)+t12.*t39.*(t289-t476+t171.*(t60-t190)).*8.084033333333334e-4))-qd5.*(qd2.*t2332+qd3.*t2332+qd4.*t2332-qd5.*(et136+et137));
et148 = qdd5.*(-t1679+t25.*t2027+t1314.*(t426-t1001)+t1321.*(t443-t1013)+t8.*t29.*(-t681+t1059.*(t61-t239).*8.084033333333334e-4+t341.*(t289-t476+t171.*(t60-t190)).*8.084033333333334e-4)+t2.*t29.*t2094)+qd6.*(qd2.*t2325+qd3.*t2325+qd4.*t2325-qd5.*(et138+et139+et140))-qdd1.*(t2027+t1101.*(t426-t1001)+t1099.*(t443-t1013));
et149 = qdd6.*((t426-t1001).^2+(t443-t1013).^2+t12.*t2033+t171.*t2094+t943.^2-t132.*(-t681+t1059.*(t61-t239).*8.084033333333334e-4+t341.*(t289-t476+t171.*(t60-t190)).*8.084033333333334e-4));
et150 = -qdd4.*(-t2013-t2098+t2.*(-t681+t1059.*(t61-t239).*8.084033333333334e-4+t341.*(t289-t476+t171.*(t60-t190)).*8.084033333333334e-4)+t2.*t773.*(t426-t1001)+t8.*t773.*(t443-t1013));
et151 = -qdd3.*(-t1852-t2098+t2.*(-t681+t1059.*(t61-t239).*8.084033333333334e-4+t341.*(t289-t476+t171.*(t60-t190)).*8.084033333333334e-4)+t2.*t890.*(t426-t1001)+t8.*t890.*(t443-t1013));
et152 = -qdd2.*(-t1900-t2098+t2.*(-t681+t1059.*(t61-t239).*8.084033333333334e-4+t341.*(t289-t476+t171.*(t60-t190)).*8.084033333333334e-4)+t2.*t942.*(t426-t1001)+t8.*t942.*(t443-t1013));
et153 = qd2.*(-qd5.*(et141+et142)+qd2.*(t1956+t1965+t2029+t2302+t2305+t943.*t1495-t2.*t953.*(t426-t1001)-t8.*t953.*(t443-t1013))+qd4.*(t1570+t1614+t1618+t1956+t1965+t2029+t2302+t2305)+qd3.*(t1647+t1663+t1764+t1956+t1965+t2029+t2302+t2305))+qd3.*(qd2.*t2322+qd3.*t2322-qd5.*(et143+et144)+qd4.*(t1570+t1614+t1618+t1930+t1931+t1977+t2302+t2305))+qd4.*(-qd5.*(et145+et146)+qd4.*(t1570+t1614+t1618+t1905+t1912+t2123+t2302+t2305)+qd3.*(t1614+t1618+t1811+t1905+t1912+t2123+t2302+t2305)+qd2.*(t1614+t1618+t1891+t1905+t1912+t2123+t2302+t2305));
mt1 = [qdd1.*(t15.*4.0513225e-3+t17.*4.0513225e-3+1.450440833333333e-3),0.0,0.0,0.0,0.0,0.0,-qd2.^2.*(t75.*t251+t71.*t259)-qdd2.*t674+qdd1.*(t18.*3.1312e-2+t3.^2.*3.1312e-2+t251.^2+t259.^2)-qd1.*qd2.*(t9.*t277.*(1.53e+2./1.25e+2)-t9.*t297.*(1.53e+2./1.25e+2))];
mt2 = [t127-qd1.*(qd2.*t667-qd1.*(t9.*t277.*(1.53e+2./2.5e+2)-t79.*t259))-qdd1.*t674+qdd2.*(t211+t212+t15.*t18.*3.74544e-1+t17.*t18.*3.74544e-1+t536.^2)+qd2.*(qd1.*t667+qd2.*(-t536.*(t15.*t63+t17.*t63)+t3.*t9.*t15.*3.74544e-1+t3.*t9.*t17.*3.74544e-1)),0.0,0.0,0.0,0.0];
mt3 = [-qdd3.*t981-qdd2.*t1128-qd2.*(t998+qd2.*(t2.*t274.*t406+t8.*t274.*t400))-qd1.*(qd2.*((t146.*t433)./5.0e+3-(t146.*t448)./5.0e+3)+qd3.*(t22.*t433.*1.1446-t22.*t448.*1.1446))+qdd1.*(t31.*2.739394083333334e-2+t20.^2.*2.739394083333334e-2+t400.^2+t406.^2)-qd3.*(t998+qd2.*t987),et14+et15,et36+et37,0.0,0.0,0.0,et1+et2];
mt4 = [et16+et17,et38+et39,et59+et60,0.0,0.0,et5+et6,et20+et21+et22,et42+et43+et44+et45,et63+et64+et65,et85+et86,0.0,et10+et11+et12+et13,et32+et33+et34+et35,et55+et56+et57+et58,et78+et79+et80,et133+et134+et135,et147+et148+et149+et150+et151+et152+et153];
Y = reshape([mt1,mt2,mt3,mt4],6,6);
end
